simulink model "InverseDynamicsControl"  (R2021a)
settings: Solver=FixedStepAuto  StartTime=0.0  StopTime=5  FixedStep=0.001  RelTol=1e-3
InitFcn:
  | Kp = [1 0 0; 0 1 0; 0 0 1];
  | Kd = [1 0 0; 0 1 0; 0 0 1];
settings Model: Creator=negin  LastModifiedBy=negin

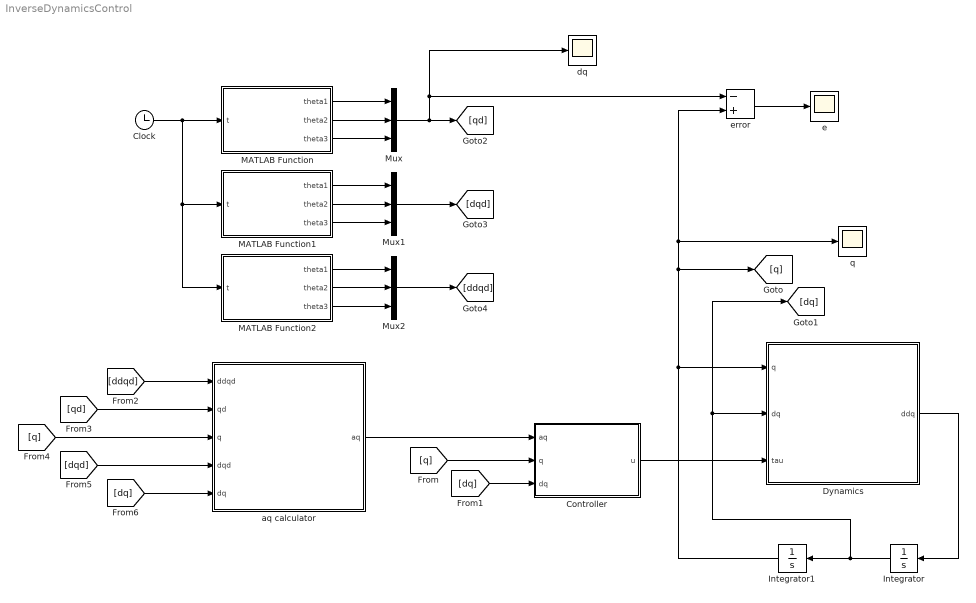
== system InverseDynamicsControl ==
  Clock : Clock
      settings: Decimation=5
  Controller : Subsystem
  Dynamics : MATLAB Function  TreatAsAtomicUnit=on
  Integrator : Integrator  InitialCondition=[0; 0; 0]
  Integrator1 : Integrator  InitialCondition=[0; 0; 0]
  MATLAB Function : MATLAB Function  TreatAsAtomicUnit=on
  MATLAB Function1 : MATLAB Function  TreatAsAtomicUnit=on
  MATLAB Function2 : MATLAB Function  TreatAsAtomicUnit=on
  Mux : Mux  Inputs=3
  Mux1 : Mux  Inputs=3
  Mux2 : Mux  Inputs=3
  aq calculator : Subsystem
  dq : Scope
  e : Scope
  error : Sum  Inputs=-+
  q : Scope
  wires:
  Dynamics/1(ddq) -> Integrator/1
  Integrator/1 -> Dynamics/2(dq), [dq], Integrator1/1
  Integrator1/1 -> Dynamics/1(q), [q], error/2, q/1
  MATLAB Function/1(theta1) -> Mux/1
  Clock/1 -> MATLAB Function2/1(t), MATLAB Function1/1(t), MATLAB Function/1(t)
  MATLAB Function/2(theta2) -> Mux/2
  MATLAB Function/3(theta3) -> Mux/3
  Mux/1 -> dq/1, error/1, [qd]
  aq calculator/1(aq) -> Controller/1(aq)
  Controller/1(u) -> Dynamics/3(tau)
  [q] -> Controller/2(q)
  MATLAB Function1/1(theta1) -> Mux1/1
  MATLAB Function1/2(theta2) -> Mux1/2
  MATLAB Function1/3(theta3) -> Mux1/3
  MATLAB Function2/1(theta1) -> Mux2/1
  MATLAB Function2/2(theta2) -> Mux2/2
  MATLAB Function2/3(theta3) -> Mux2/3
  Mux1/1 -> [dqd]
  Mux2/1 -> [ddqd]
  [ddqd] -> aq calculator/1(ddqd)
  [qd] -> aq calculator/2(qd)
  [q] -> aq calculator/3(q)
  [dqd] -> aq calculator/4(dqd)
  [dq] -> aq calculator/5(dq)
  [dq] -> Controller/3(dq)
  error/1 -> e/1

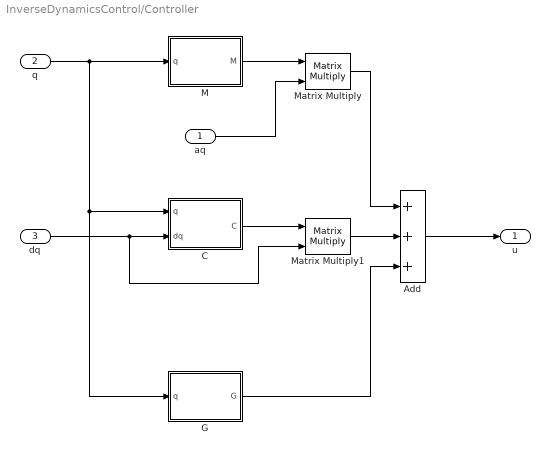
== system InverseDynamicsControl/Controller ==
  aq : Inport
  q : Inport  Port=2
  dq : Inport  Port=3
  Add : Sum  Inputs=+++
  C : MATLAB Function  TreatAsAtomicUnit=on
  G : MATLAB Function  TreatAsAtomicUnit=on
  M : MATLAB Function  TreatAsAtomicUnit=on
  Matrix Multiply : Product  Multiplication=Matrix(*)
  Matrix Multiply1 : Product  Multiplication=Matrix(*)
  u : Outport
  wires:
  q/1 -> M/1(q), C/1(q), G/1(q)
  aq/1 -> Matrix Multiply/2
  dq/1 -> Matrix Multiply1/2, C/2(dq)
  M/1(M) -> Matrix Multiply/1
  Matrix Multiply/1 -> Add/1
  G/1(G) -> Add/3
  Add/1 -> u/1
  C/1(C) -> Matrix Multiply1/1
  Matrix Multiply1/1 -> Add/2

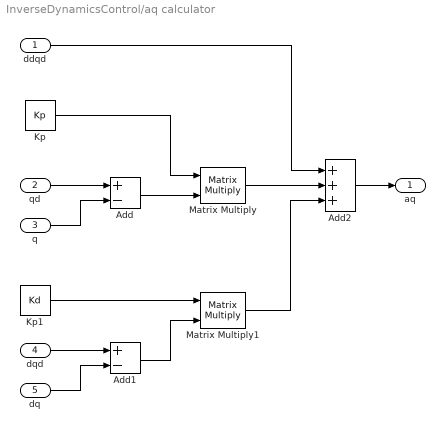
== system InverseDynamicsControl/aq calculator ==
  ddqd : Inport
  qd : Inport  Port=2
  q : Inport  Port=3
  dqd : Inport  Port=4
  dq : Inport  Port=5
  Add : Sum  Inputs=+-
  Add1 : Sum  Inputs=+-
  Add2 : Sum  Inputs=+++
  Kp : Constant  Value=Kp
  Kp1 : Constant  Value=Kd
  Matrix Multiply : Product  Multiplication=Matrix(*)
  Matrix Multiply1 : Product  Multiplication=Matrix(*)
  aq : Outport
  wires:
  qd/1 -> Add/1
  q/1 -> Add/2
  dqd/1 -> Add1/1
  dq/1 -> Add1/2
  Add/1 -> Matrix Multiply/2
  Kp/1 -> Matrix Multiply/1
  Kp1/1 -> Matrix Multiply1/1
  Add1/1 -> Matrix Multiply1/2
  Matrix Multiply/1 -> Add2/2
  Matrix Multiply1/1 -> Add2/3
  ddqd/1 -> Add2/1
  Add2/1 -> aq/1

== matlab function InverseDynamicsControl/MATLAB Function ==
  data: theta1 output; t input; theta2 output; theta3 output
function [theta1, theta2, theta3] = desiredTraj(t)
theta1 = 0.1309*t^2 + 0.0147*t^3 - 0.0085*t^4 + 0.0007*t^5;
theta2 = 0.1309*t^2 - 0.0188*t^3 - 0.001*t^4 + 0.0002*t^5;
theta3 = 0.1309*t^2 + 0.0314*t^3 - 0.0123*t^4 + 0.001*t^5;

== matlab function InverseDynamicsControl/Dynamics ==
  data: q input; ddq output; dq input; tau input
function ddq = RobotDynamics(q, dq, tau)

m1 = 1;
m2 = 1;
m3 = 1;

l1 = 1;
l2 = 1;
l3 = 1;

r1 = l1/2;
r2 = l2/2;
r3 = l3/2;

R1 = 0.05;
R2 = 0.05;
R3 = 0.05;

g = 9.81;

a1 = m2*r2^2 + m3*l2^2;
a2 = m3*r3^2;
a3 = m3*r3*l2;
b1 = (m2*r2 + m3*l2)*g;
b2 = m3*r3*g;
I1 = 0.5*m1*R1^2;
I2 = 0.5*m2*R2^2;
I3 = 0.5*m3*R3^2;

M11 = a1*cos(q(2))^2 + a2*cos(q(2) + q(3))^2 + 2*a3*cos(q(2))*cos(q(2) + q(3)) + I1;
M12 = 0; 
M13 = 0; 
M21 = 0; 
M31 = 0;
M22 = a1 + a2 + 2*a3*cos(q(3)) + I2;
M23 = a2 + a3*cos(q(3));
M32 = a2 + a3*cos(q(3));
M33 = a2 + I3;
M = [M11 M12 M13; M21 M22 M23; M31 M32 M33];

C11 = -0.5*a1*dq(2)*sin(2*q(2)) - 0.5*a2*(dq(2) + dq(3))*sin(2*q(2) + 2*q(3))...
    - a3*dq(2)*sin(2*q(2) + q(3)) - a3*dq(3)*cos(q(2))*sin(q(2) + q(3));
C12 = -0.5*a1*dq(1)*sin(2*q(2)) - 0.5*a2*dq(1)*sin(2*q(2) + 2*q(3)) - ...
    a3*dq(1)*sin(2*q(2) + q(3));
C13 = -0.5*a2*dq(1)*sin(2*q(2) + 2*q(3)) - a3*dq(1)*cos(q(2))*sin(q(2) + q(3));
C21 = -C12;
C22 = -a3*dq(3)*sin(q(3));
C23 = -a3*(dq(2) + dq(3))*sin(q(3));
C31 = -C13;
C32 = a3*dq(2)*sin(q(3));
C33 = 0;
C = [C11 C12 C13; C21 C22 C23; C31 C32 C33];

G11 = 0;
G21 = m2*l2*sin(q(2))*g/2 - m3*l3*sin(q(2) + q(3))*g/2 - m3*l2*sin(q(2))*g;
G31 = -m3*l3*sin(q(2) + q(3))*g/2;
G = [G11; G21; G31];

ddq = inv(M)*(tau - C*dq - G);
end

== matlab function InverseDynamicsControl/Controller/M ==
  data: q input; M output
function M = Mmatrix(q)

m1 = 1;
m2 = 1;
m3 = 1;

l1 = 1;
l2 = 1;
l3 = 1;

r1 = l1/2;
r2 = l2/2;
r3 = l3/2;

R1 = 0.05;
R2 = 0.05;
R3 = 0.05;

g = 9.81;

a1 = m2*r2^2 + m3*l2^2;
a2 = m3*r3^2;
a3 = m3*r3*l2;
b1 = (m2*r2 + m3*l2)*g;
b2 = m3*r3*g;
I1 = 0.5*m1*R1^2;
I2 = 0.5*m2*R2^2;
I3 = 0.5*m3*R3^2;

M11 = a1*cos(q(2))^2 + a2*cos(q(2) + q(3))^2 + 2*a3*cos(q(2))*cos(q(2) + q(3)) + I1;
M12 = 0; 
M13 = 0; 
M21 = 0; 
M31 = 0;
M22 = a1 + a2 + 2*a3*cos(q(3)) + I2;
M23 = a2 + a3*cos(q(3));
M32 = a2 + a3*cos(q(3));
M33 = a2 + I3;
M = [M11 M12 M13; M21 M22 M23; M31 M32 M33];

end

== matlab function InverseDynamicsControl/Controller/C ==
  data: q input; C output; dq input
function C = Cmatrix(q, dq)

m1 = 1;
m2 = 1;
m3 = 1;

l1 = 1;
l2 = 1;
l3 = 1;

r1 = l1/2;
r2 = l2/2;
r3 = l3/2;

R1 = 0.05;
R2 = 0.05;
R3 = 0.05;

g = 9.81;

a1 = m2*r2^2 + m3*l2^2;
a2 = m3*r3^2;
a3 = m3*r3*l2;
b1 = (m2*r2 + m3*l2)*g;
b2 = m3*r3*g;
I1 = 0.5*m1*R1^2;
I2 = 0.5*m2*R2^2;
I3 = 0.5*m3*R3^2;

C11 = -0.5*a1*dq(2)*sin(2*q(2)) - 0.5*a2*(dq(2) + dq(3))*sin(2*q(2) + 2*q(3))...
    - a3*dq(2)*sin(2*q(2) + q(3)) - a3*dq(3)*cos(q(2))*sin(q(2) + q(3));
C12 = -0.5*a1*dq(1)*sin(2*q(2)) - 0.5*a2*dq(1)*sin(2*q(2) + 2*q(3)) - ...
    a3*dq(1)*sin(2*q(2) + q(3));
C13 = -0.5*a2*dq(1)*sin(2*q(2) + 2*q(3)) - a3*dq(1)*cos(q(2))*sin(q(2) + q(3));
C21 = -C12;
C22 = -a3*dq(3)*sin(q(3));
C23 = -a3*(dq(2) + dq(3))*sin(q(3));
C31 = -C13;
C32 = a3*dq(2)*sin(q(3));
C33 = 0;
C = [C11 C12 C13; C21 C22 C23; C31 C32 C33];

end

== matlab function InverseDynamicsControl/Controller/G ==
  data: q input; G output
function G = Gmatrix(q)

m1 = 1;
m2 = 1;
m3 = 1;

l1 = 1;
l2 = 1;
l3 = 1;

r1 = l1/2;
r2 = l2/2;
r3 = l3/2;

R1 = 0.05;
R2 = 0.05;
R3 = 0.05;

g = 9.81;

a1 = m2*r2^2 + m3*l2^2;
a2 = m3*r3^2;
a3 = m3*r3*l2;
b1 = (m2*r2 + m3*l2)*g;
b2 = m3*r3*g;
I1 = 0.5*m1*R1^2;
I2 = 0.5*m2*R2^2;
I3 = 0.5*m3*R3^2;

G11 = 0;
G21 = m2*l2*sin(q(2))*g/2 - m3*l3*sin(q(2) + q(3))*g/2 - m3*l2*sin(q(2))*g;
G31 = -m3*l3*sin(q(2) + q(3))*g/2;
G = [G11; G21; G31];

end

== matlab function InverseDynamicsControl/MATLAB Function1 ==
  data: theta1 output; t input; theta2 output; theta3 output
function [theta1, theta2, theta3] = ddesiredTraj(t)
theta1 = 0.1309*2*t + 0.0147*3*t^2 - 0.0085*4*t^3 + 0.0007*5*t^4;
theta2 = 0.1309*2*t - 0.0188*3*t^2 - 0.001*4*t^3 + 0.0002*5*t^4;
theta3 = 0.1309*2*t + 0.0314*3*t^2 - 0.0123*4*t^3 + 0.001*5*t^4;

== matlab function InverseDynamicsControl/MATLAB Function2 ==
  data: theta1 output; t input; theta2 output; theta3 output
function [theta1, theta2, theta3] = dddesiredTraj(t)
theta1 = 0.1309*2 + 0.0147*3*2*t - 0.0085*4*3*t^2 + 0.0007*5*4*t^3;
theta2 = 0.1309*2 - 0.0188*3*2*t - 0.001*4*3*t^2 + 0.0002*5*4*t^3;
theta3 = 0.1309*2 + 0.0314*3*2*t - 0.0123*4*3*t^2 + 0.001*5*4*t^3;
